simulink model "FLC_MCC"  (Simulink 8.5)
settings: Solver=ode5  StartTime=0.0  StopTime=2  FixedStep=0.0001  RelTol=1e-3
libraries: fuzblock x1
settings Model: Creator=areerees  LastModifiedBy=USER
settings OptimizationCC: InitFltsAndDblsToZero=on
settings DebuggingCC: SolverPrmCheckMsg=warning  FcnCallInpInsideContextMsg=UseLocalSettings

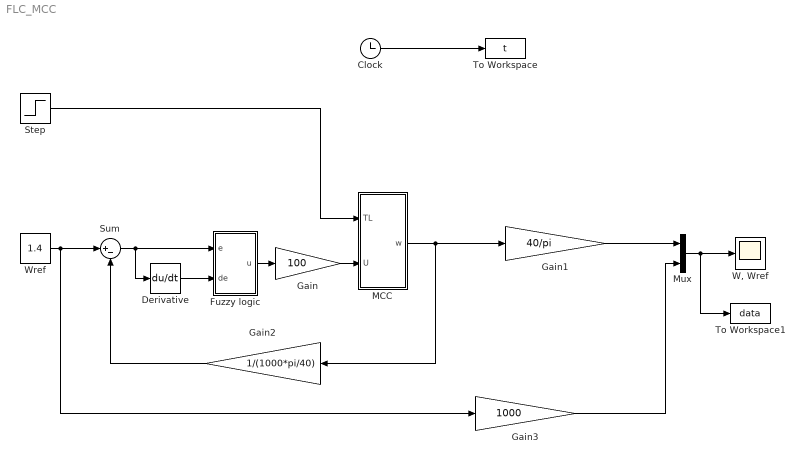
== system FLC_MCC ==
  Clock : Clock
  Derivative : Derivative
  Fuzzy logic : Subsystem  mask{Ge=2, Gde=0.1, Gdu=19}
      mask Display: disp('clf')
  Gain : Gain  Gain=100
  Gain1 : Gain  Gain=40/pi
  Gain2 : Gain  Gain=1/(1000*pi/40)
  Gain3 : Gain  Gain=1000
  MCC : Subsystem  mask{Kv=0.91, If=1.4, Rm=0.1, Lm=0.0001, J=0.01, B=0.3}
      mask Display: disp('MCC')
  Mux : Mux  Inputs=2
  Step : Step  Before=10  After=12  SampleTime=0
  Sum : Sum  Inputs=|+-
  To Workspace : ToWorkspace  VariableName=t  SampleTime=-1
  To Workspace1 : ToWorkspace  VariableName=data  SampleTime=-1
  "W, Wref" : Scope
      settings: YMin=0  YMax=1500
  Wref : Constant  Value=1.4
  wires:
  MCC/1(w) -> Gain1/1, Gain2/1
  Fuzzy logic/1(u) -> Gain/1
  Wref/1 -> Sum/1, Gain3/1
  Sum/1 -> Fuzzy logic/1(e), Derivative/1
  Derivative/1 -> Fuzzy logic/2(de)
  Step/1 -> MCC/1(TL)
  Mux/1 -> "W, Wref"/1, To Workspace1/1
  Clock/1 -> To Workspace/1
  Gain/1 -> MCC/2(U)
  Gain3/1 -> Mux/2
  Gain1/1 -> Mux/1
  Gain2/1 -> Sum/2

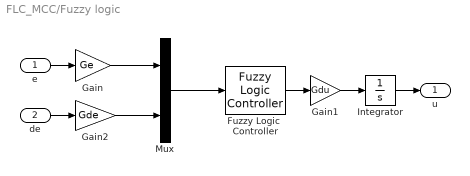
== system FLC_MCC/Fuzzy logic ==
  e : Inport
  de : Inport  Port=2
  Fuzzy Logic  Controller : fuzblock/Fuzzy Logic  Controller  fis='Fuzzy_FIS.fis'
  Gain : Gain  Gain=Ge
  Gain1 : Gain  Gain=Gdu
  Gain2 : Gain  Gain=Gde
  Integrator : Integrator
  Mux : Mux  Inputs=2
  u : Outport
  wires:
  Gain1/1 -> Integrator/1
  Fuzzy Logic  Controller/1 -> Gain1/1
  Mux/1 -> Fuzzy Logic  Controller/1
  Gain2/1 -> Mux/2
  Gain/1 -> Mux/1
  e/1 -> Gain/1
  Integrator/1 -> u/1
  de/1 -> Gain2/1

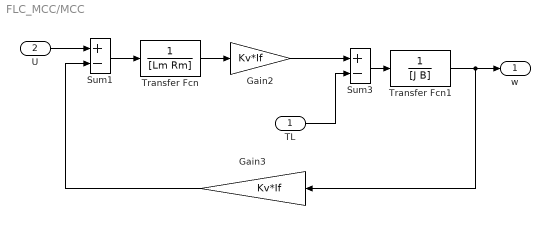
== system FLC_MCC/MCC ==
  TL : Inport
  U : Inport  Port=2
  Gain2 : Gain  Gain=Kv*If
  Gain3 : Gain  Gain=Kv*If
  Sum1 : Sum  Inputs=+-
  Sum3 : Sum  Inputs=+-
  Transfer Fcn : TransferFcn  Denominator=[Lm Rm]
  Transfer Fcn1 : TransferFcn  Denominator=[J B]
  w : Outport
  wires:
  Transfer Fcn/1 -> Gain2/1
  Gain2/1 -> Sum3/1
  Transfer Fcn1/1 -> Gain3/1, w/1
  Sum1/1 -> Transfer Fcn/1
  Gain3/1 -> Sum1/2
  TL/1 -> Sum3/2
  Sum3/1 -> Transfer Fcn1/1
  U/1 -> Sum1/1
